simulink model "MBD_Prob6"  (R2020a)
settings: Solver=VariableStepAuto  StartTime=0.0  StopTime=10.0  RelTol=1e-3
settings Model: Creator=Noel Varghese  LastModifiedBy=Noel Varghese

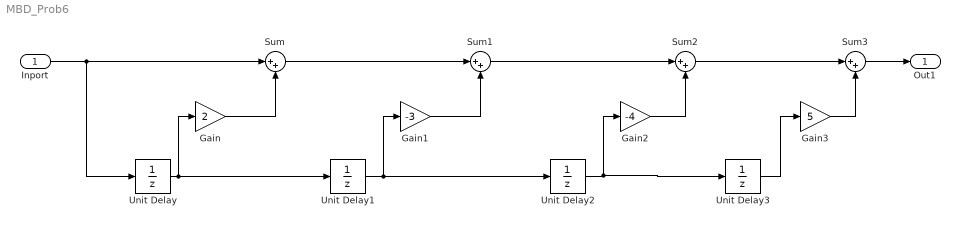
== system MBD_Prob6 ==
  Inport : Inport
  Gain : Gain  Gain=2
  Gain1 : Gain  Gain=-3
  Gain2 : Gain  Gain=-4
  Gain3 : Gain  Gain=5
  Sum{,1..3} (4 alike) : Sum  Inputs=|++
  Unit Delay{,1..3} (4 alike) : UnitDelay  SampleTime=-1  HasFrameUpgradeWarning=on
  Out1 : Outport
  wires:
  Unit Delay/1 -> Unit Delay1/1, Gain/1
  Gain/1 -> Sum/2
  Unit Delay1/1 -> Unit Delay2/1, Gain1/1
  Gain1/1 -> Sum1/2
  Gain2/1 -> Sum2/2
  Unit Delay2/1 -> Unit Delay3/1, Gain2/1
  Unit Delay3/1 -> Gain3/1
  Gain3/1 -> Sum3/2
  Inport/1 -> Unit Delay/1, Sum/1
  Sum/1 -> Sum1/1
  Sum1/1 -> Sum2/1
  Sum2/1 -> Sum3/1
  Sum3/1 -> Out1/1
